simulink model "P60"  (R2015b)
settings: Solver=VariableStepAuto  StartTime=0.0  StopTime=10.0  RelTol=1e-3
settings Model: Creator=xmax1946  LastModifiedBy=xmax1946

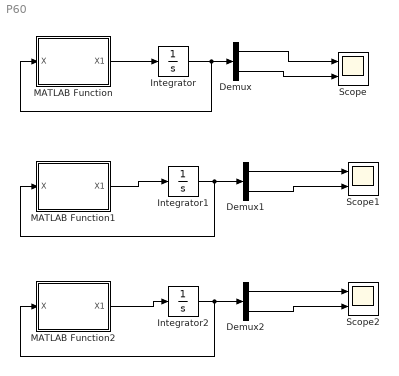
== system P60 ==
  Demux : Demux  Outputs=2
  Demux1 : Demux  Outputs=2
  Demux2 : Demux  Outputs=2
  Integrator : Integrator  InitialCondition=[0;0]
  Integrator1 : Integrator  InitialCondition=[0;0]
  Integrator2 : Integrator  InitialCondition=[0;0]
  MATLAB Function : MATLAB Function  TreatAsAtomicUnit=on
  MATLAB Function1 : MATLAB Function  TreatAsAtomicUnit=on
  MATLAB Function2 : MATLAB Function  TreatAsAtomicUnit=on
  Scope : Scope  NumInputPorts=2
  Scope1 : Scope  NumInputPorts=2
  Scope2 : Scope  NumInputPorts=2
  wires:
  MATLAB Function/1(X1) -> Integrator/1
  Integrator/1 -> MATLAB Function/1(X), Demux/1
  Integrator1/1 -> MATLAB Function1/1(X), Demux1/1
  Demux/1 -> Scope/1
  Demux/2 -> Scope/2
  Demux1/1 -> Scope1/1
  Demux1/2 -> Scope1/2
  MATLAB Function1/1(X1) -> Integrator1/1
  Integrator2/1 -> MATLAB Function2/1(X), Demux2/1
  Demux2/1 -> Scope2/1
  Demux2/2 -> Scope2/2
  MATLAB Function2/1(X1) -> Integrator2/1

== matlab function P60/MATLAB Function1 ==
  data: X input; X1 output
function X1 = fcn(X)
r=1;
K=[4,14/3];
u=r-K*X;
A=[1,3;3,1];
B=[1;0];
X1=A*X+B*u;

== matlab function P60/MATLAB Function ==
  data: X input; X1 output
function X1 = fcn(X)
u=1;
A=[1,3;3,1];
B=[1;0];
X1=A*X+B*u;

== matlab function P60/MATLAB Function2 ==
  data: X input; X1 output
function X1 = fcn(X)
r=1;
K=[3.5,4];
u=r-K*X;
A=[1,3;3,1];
B=[1;0];
X1=A*X+B*u;
